simulink model "ROV"  (R2018a)
settings: Solver=FixedStepAuto  StartTime=0.0  StopTime=inf  RelTol=1e-3  EnableMultiTasking=on
libraries: embdlinuxlib x1
settings Model: Creator=RHughes  LastModifiedBy=RHughes
settings SolverCC: PositivePriorityOrder=on
settings OptimizationCC: PassReuseOutputArgsThreshold=0  MaxStackSize=64
settings DebuggingCC: ParameterTunabilityLossMsg=error
settings HardwareCC: ProdBitPerPointer=32  ProdBitPerSizeT=32  ProdBitPerPtrDiffT=32  ProdLargestAtomicInteger=Long  ProdLargestAtomicFloat=Double  ProdWordSize=32  ProdHWDeviceType=ARM Compatible->ARM Cortex  UseEmbeddedCoderFeatures=off
settings SFSimCC: MATLABDynamicMemAlloc=off
settings RTWCC: SystemTargetFile=ert.tlc  HardwareBoard=Raspberry Pi  TLCOptions="-aInlineSetEventsForThisBaseRateFcn=TLC_FALSE -aSuppressMultiTaskScheduler=TLC_FALSE  -aRateBasedStepFcn=0"  TemplateMakefile=ert_default_tmf  GenerateReport=on  Toolchain=GNU GCC Raspberry Pi  LaunchReport=on
settings CodeAppCC: ForceParamTrailComments=on  OperatorAnnotations=on
settings ERTTargetCC: ERTCustomFileBanners=off  SupportContinuousTime=on  SupportNonInlinedSFcns=on  RemoveResetFunc=off  SupportVariableSizeSignals=on  ModelStepFunctionPrototypeControlCompliant=off

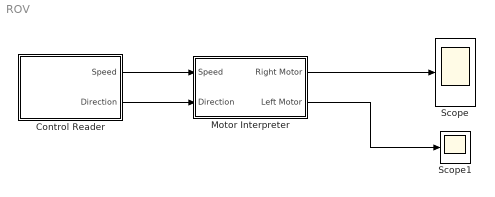
== system ROV ==
  Control Reader : Subsystem
  Motor Interpreter : Subsystem
  Scope : Scope
  Scope1 : Scope
  wires:
  Control Reader/1(Speed) -> Motor Interpreter/1("Speed ")
  Control Reader/2(Direction) -> Motor Interpreter/2(Direction)
  Motor Interpreter/1(Right Motor) -> Scope/1
  Motor Interpreter/2(Left Motor) -> Scope1/1

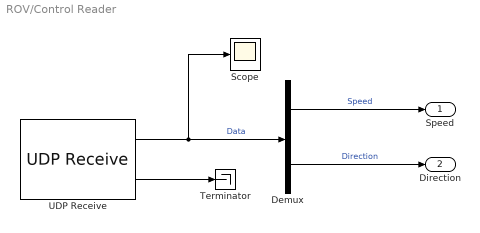
== system ROV/Control Reader ==
  Demux : Demux  Outputs=2
  Scope : Scope
  Terminator : Terminator
  UDP Receive : embdlinuxlib/UDP Receive  localURL='0.0.0.0'  localPort=25000  remoteURL='0.0.0.0'  remotePort=-1  recvBufferSize=8192  signalDatatype=int8  dims=2  isVarSize=off  showBlockingTime=off  blockingTime=0  sampletime=0.01  blockPlatform=Raspberry Pi
      settings: SourceProductName=Simulink Support Package for Raspberry Pi Hardware  SourceProductBaseCode=RASPPI
  Speed : Outport
  Direction : Outport  Port=2
  wires:
  Demux/1 -> Speed/1  "Speed"
  Demux/2 -> Direction/1  "Direction"
  UDP Receive/1 -> Scope/1, Demux/1  "Data"
  UDP Receive/2 -> Terminator/1

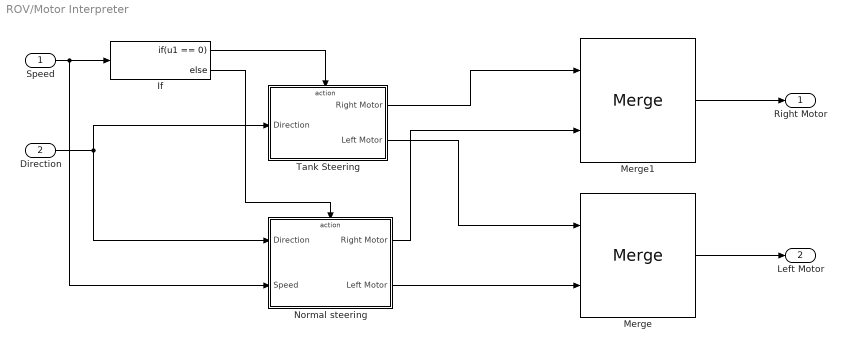
== system ROV/Motor Interpreter ==
  "Speed " : Inport
  Direction : Inport  Port=2
  If : If  IfExpression=u1 == 0
  Merge : Merge
  Merge1 : Merge
  Normal steering : Subsystem  TreatAsAtomicUnit=on
  Tank Steering : Subsystem  TreatAsAtomicUnit=on
  Right Motor : Outport
  Left Motor : Outport  Port=2
  wires:
  If/1 -> Tank Steering/Action
  "Speed "/1 -> Normal steering/2(Speed), If/1
  Direction/1 -> Normal steering/1(Direction), Tank Steering/1("Direction ")
  If/2 -> Normal steering/Action
  Tank Steering/2(Left Motor) -> Merge/1
  Normal steering/2(Left Motor) -> Merge/2
  Normal steering/1(Right Motor) -> Merge1/2
  Tank Steering/1(Right Motor) -> Merge1/1
  Merge/1 -> Left Motor/1
  Merge1/1 -> Right Motor/1

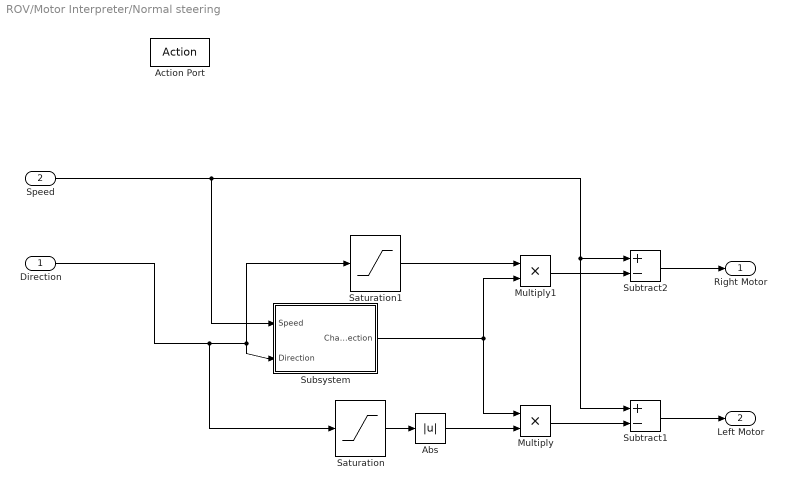
== system ROV/Motor Interpreter/Normal steering ==
  Direction : Inport
  Speed : Inport  Port=2
  Action Port : ActionPort  ActionType=else
  Abs : Abs
  Multiply : Product  OutDataTypeStr=int8
  Multiply1 : Product  OutDataTypeStr=int8
  Saturation : Saturate  UpperLimit=0  LowerLimit=-1  LinearizeAsGain=off
  Saturation1 : Saturate  UpperLimit=1  LowerLimit=0
  Subsystem : Subsystem
  Subtract1 : Sum  Inputs=+-  AccumDataTypeStr=int8
  Subtract2 : Sum  Inputs=+-  AccumDataTypeStr=int8
  Right Motor : Outport
  Left Motor : Outport  Port=2
  wires:
  Direction/1 -> Saturation1/1, Subsystem/2(Direction), Saturation/1
  Saturation1/1 -> Multiply1/1
  Multiply1/1 -> Subtract2/2
  Subtract2/1 -> Right Motor/1
  Saturation/1 -> Abs/1
  Subtract1/1 -> Left Motor/1
  Abs/1 -> Multiply/2
  Multiply/1 -> Subtract1/2
  Subsystem/1(Change_in_direction) -> Multiply1/2, Multiply/1
  Speed/1 -> Subtract1/1, Subtract2/1, Subsystem/1(Speed)

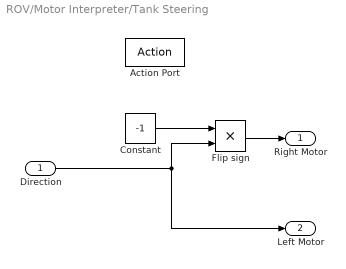
== system ROV/Motor Interpreter/Tank Steering ==
  "Direction " : Inport
  Action Port : ActionPort  ActionType=then
  Constant : Constant  Value=-1  OutDataTypeStr=int8
  Flip sign : Product  OutDataTypeStr=int8
  Right Motor : Outport
  Left Motor : Outport  Port=2  OutDataTypeStr=int8
  wires:
  "Direction "/1 -> Flip sign/2, Left Motor/1
  Flip sign/1 -> Right Motor/1
  Constant/1 -> Flip sign/1

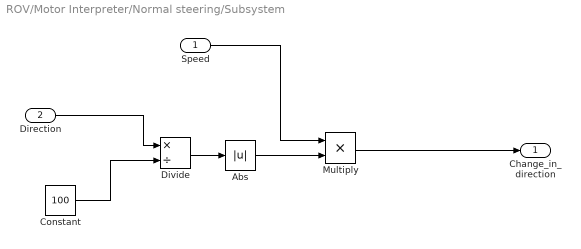
== system ROV/Motor Interpreter/Normal steering/Subsystem ==
  Speed : Inport
  Direction : Inport  Port=2
  Abs : Abs
  Constant : Constant  Value=100  OutDataTypeStr=int8
  Divide : Product  Inputs=*/
  Multiply : Product  OutDataTypeStr=int8
  Change_in_direction : Outport
  wires:
  Direction/1 -> Divide/1
  Constant/1 -> Divide/2
  Speed/1 -> Multiply/1
  Divide/1 -> Abs/1
  Abs/1 -> Multiply/2
  Multiply/1 -> Change_in_direction/1
